simulink model "HANcoder_E407_TTA_Template_DS_V61"  (R2023a)
settings: Solver=FixedStepDiscrete  StartTime=0.0  StopTime=1  FixedStep=0.01  RelTol=1e-3
PreLoadFcn:
  | librarySetup
  | eval([bdroot,'_startup']) %Calling [modelName]_startup.m
values from neighbouring files (symbols this model uses):
  basic_cycle_duration_bc0 = TM_Reset_Board   + COMP_duration    (= 372)    [HANcoder_E407_TTA_Template_DS_V1_startup.m]    (also in HANcoder_E407_TTA_Template_DS_V2_startup.m; HANcoder_E407_TTA_Template_DS_V52_startup.m; HANcoder_E407_TTA_Template_DS_V5_startup.m; HANcoder_E407_TTA_Template_DS_V6_startup.m = 532)
  basic_cycle_duration_bc1 = basic_cycle_duration_bc0    (= 372)    [HANcoder_E407_TTA_Template_DS_V1_startup.m]    (also in HANcoder_E407_TTA_Template_DS_V2_startup.m; HANcoder_E407_TTA_Template_DS_V52_startup.m; HANcoder_E407_TTA_Template_DS_V5_startup.m; HANcoder_E407_TTA_Template_DS_V6_startup.m = 532)
  basic_cycle_duration_bc2 = basic_cycle_duration_bc0    (= 372)    [HANcoder_E407_TTA_Template_DS_V1_startup.m]    (also in HANcoder_E407_TTA_Template_DS_V2_startup.m; HANcoder_E407_TTA_Template_DS_V52_startup.m; HANcoder_E407_TTA_Template_DS_V5_startup.m; HANcoder_E407_TTA_Template_DS_V6_startup.m = 532)
  comm_delay_estimation1 = round(comm_delay_measured1*hardware_granularity/frequency_IRQ)    [HANcoder_E407_TTA_Template_DS_V1_startup.m]    (also in HANcoder_E407_TTA_Template_DS_V2_startup.m; HANcoder_E407_TTA_Template_DS_V52_startup.m; HANcoder_E407_TTA_Template_DS_V5_startup.m; HANcoder_E407_TTA_Template_DS_V6_startup.m)
  comm_delay_estimation2 = round(comm_delay_measured2*hardware_granularity/frequency_IRQ)    [HANcoder_E407_TTA_Template_DS_V1_startup.m]    (also in HANcoder_E407_TTA_Template_DS_V2_startup.m; HANcoder_E407_TTA_Template_DS_V52_startup.m; HANcoder_E407_TTA_Template_DS_V5_startup.m; HANcoder_E407_TTA_Template_DS_V6_startup.m)
  COMM_Period = 80    [HANcoder_E407_TTA_Template_DS_V1_startup.m]    (also in HANcoder_E407_TTA_Template_DS_V2_startup.m; HANcoder_E407_TTA_Template_DS_V52_startup.m; HANcoder_E407_TTA_Template_DS_V5_startup.m; HANcoder_E407_TTA_Template_DS_V6_startup.m = 120)
  COMM_Phase1 = Simulink.Parameter    [HANcoder_E407_TTA_Template_DS_V1_startup.m]    (also in HANcoder_E407_TTA_Template_DS_V2_startup.m; HANcoder_E407_TTA_Template_DS_V52_startup.m; HANcoder_E407_TTA_Template_DS_V5_startup.m; HANcoder_E407_TTA_Template_DS_V6_startup.m)
  COMM_Phase2 = Simulink.Parameter    [HANcoder_E407_TTA_Template_DS_V1_startup.m]    (also in HANcoder_E407_TTA_Template_DS_V2_startup.m; HANcoder_E407_TTA_Template_DS_V52_startup.m; HANcoder_E407_TTA_Template_DS_V5_startup.m; HANcoder_E407_TTA_Template_DS_V6_startup.m)
  COMM_Phase_init1 = Simulink.Parameter    [HANcoder_E407_TTA_Template_DS_V1_startup.m]    (also in HANcoder_E407_TTA_Template_DS_V2_startup.m; HANcoder_E407_TTA_Template_DS_V52_startup.m; HANcoder_E407_TTA_Template_DS_V5_startup.m; HANcoder_E407_TTA_Template_DS_V6_startup.m)
  COMM_Phase_init2 = Simulink.Parameter    [HANcoder_E407_TTA_Template_DS_V1_startup.m]    (also in HANcoder_E407_TTA_Template_DS_V2_startup.m; HANcoder_E407_TTA_Template_DS_V52_startup.m; HANcoder_E407_TTA_Template_DS_V5_startup.m; HANcoder_E407_TTA_Template_DS_V6_startup.m)
  COMP_duration = 4    [HANcoder_E407_TTA_Template_DS_V1_startup.m]    (also in HANcoder_E407_TTA_Template_DS_V2_startup.m; HANcoder_E407_TTA_Template_DS_V52_startup.m; HANcoder_E407_TTA_Template_DS_V5_startup.m; HANcoder_E407_TTA_Template_DS_V6_startup.m)
  frequency_IRQ = 100    [HANcoder_E407_TTA_Template_DS_V1_startup.m]    (also in HANcoder_E407_TTA_Template_DS_V2_startup.m; HANcoder_E407_TTA_Template_DS_V52_startup.m; HANcoder_E407_TTA_Template_DS_V5_startup.m; HANcoder_E407_TTA_Template_DS_V6_startup.m)
  idle_time_init = basic_cycle_duration_bc0 + basic_cycle_duration_bc1    (= 744)    [HANcoder_E407_TTA_Template_DS_V1_startup.m]    (also in HANcoder_E407_TTA_Template_DS_V2_startup.m; HANcoder_E407_TTA_Template_DS_V52_startup.m = 1116; HANcoder_E407_TTA_Template_DS_V5_startup.m = 1116; HANcoder_E407_TTA_Template_DS_V6_startup.m = 1596)
  L0b = 0.5    [HANcoder_E407_TTA_Template_DS_V52_startup.m]    (also in HANcoder_E407_TTA_Template_DS_V5_startup.m; HANcoder_E407_TTA_Template_DS_V6_startup.m)
  L0f = 5    [HANcoder_E407_TTA_Template_DS_V52_startup.m]    (also in HANcoder_E407_TTA_Template_DS_V5_startup.m; HANcoder_E407_TTA_Template_DS_V6_startup.m)
  L1f = 6    [HANcoder_E407_TTA_Template_DS_V52_startup.m]    (also in HANcoder_E407_TTA_Template_DS_V5_startup.m; HANcoder_E407_TTA_Template_DS_V6_startup.m)
  LA_Clock_Gr = 1    [HANcoder_E407_TTA_Template_DS_V1_startup.m]    (also in HANcoder_E407_TTA_Template_DS_V2_startup.m; HANcoder_E407_TTA_Template_DS_V52_startup.m; HANcoder_E407_TTA_Template_DS_V5_startup.m; HANcoder_E407_TTA_Template_DS_V6_startup.m)
  LA_COMM_dly = 1    [HANcoder_E407_TTA_Template_DS_V1_startup.m]    (also in HANcoder_E407_TTA_Template_DS_V2_startup.m; HANcoder_E407_TTA_Template_DS_V52_startup.m; HANcoder_E407_TTA_Template_DS_V5_startup.m; HANcoder_E407_TTA_Template_DS_V6_startup.m)
  LA_COMM_Err = 1    [HANcoder_E407_TTA_Template_DS_V1_startup.m]    (also in HANcoder_E407_TTA_Template_DS_V2_startup.m; HANcoder_E407_TTA_Template_DS_V52_startup.m; HANcoder_E407_TTA_Template_DS_V5_startup.m; HANcoder_E407_TTA_Template_DS_V6_startup.m)
  LA_E_Desync = 1    [HANcoder_E407_TTA_Template_DS_V1_startup.m]    (also in HANcoder_E407_TTA_Template_DS_V2_startup.m; HANcoder_E407_TTA_Template_DS_V52_startup.m; HANcoder_E407_TTA_Template_DS_V5_startup.m; HANcoder_E407_TTA_Template_DS_V6_startup.m)
  LA_MEX_Flag = 1    [HANcoder_E407_TTA_Template_DS_V1_startup.m]    (also in HANcoder_E407_TTA_Template_DS_V2_startup.m; HANcoder_E407_TTA_Template_DS_V52_startup.m; HANcoder_E407_TTA_Template_DS_V5_startup.m; HANcoder_E407_TTA_Template_DS_V6_startup.m)
  LA_Task_Act = 1    [HANcoder_E407_TTA_Template_DS_V1_startup.m]    (also in HANcoder_E407_TTA_Template_DS_V2_startup.m; HANcoder_E407_TTA_Template_DS_V52_startup.m; HANcoder_E407_TTA_Template_DS_V5_startup.m; HANcoder_E407_TTA_Template_DS_V6_startup.m)
  Master_Role = 1    [HANcoder_E407_TTA_Template_DS_V1_startup.m]    (also in HANcoder_E407_TTA_Template_DS_V2_startup.m; HANcoder_E407_TTA_Template_DS_V52_startup.m; HANcoder_E407_TTA_Template_DS_V5_startup.m; HANcoder_E407_TTA_Template_DS_V6_startup.m)
  matrix_rows = 3    [HANcoder_E407_TTA_Template_DS_V1_startup.m]    (also in HANcoder_E407_TTA_Template_DS_V2_startup.m; HANcoder_E407_TTA_Template_DS_V52_startup.m; HANcoder_E407_TTA_Template_DS_V5_startup.m; HANcoder_E407_TTA_Template_DS_V6_startup.m)
  max_desync = 15    [HANcoder_E407_TTA_Template_DS_V1_startup.m]    (also in HANcoder_E407_TTA_Template_DS_V2_startup.m; HANcoder_E407_TTA_Template_DS_V52_startup.m; HANcoder_E407_TTA_Template_DS_V5_startup.m; HANcoder_E407_TTA_Template_DS_V6_startup.m)
  max_num_msgs_CAN1 = 2^Tx_bit_number-1    (= 7)    [HANcoder_E407_TTA_Template_DS_V1_startup.m]    (also in HANcoder_E407_TTA_Template_DS_V2_startup.m; HANcoder_E407_TTA_Template_DS_V52_startup.m; HANcoder_E407_TTA_Template_DS_V5_startup.m; HANcoder_E407_TTA_Template_DS_V6_startup.m)
  max_num_msgs_CAN2 = max_num_msgs_CAN1    (= 7)    [HANcoder_E407_TTA_Template_DS_V1_startup.m]    (also in HANcoder_E407_TTA_Template_DS_V2_startup.m; HANcoder_E407_TTA_Template_DS_V52_startup.m; HANcoder_E407_TTA_Template_DS_V5_startup.m; HANcoder_E407_TTA_Template_DS_V6_startup.m)
  min_desync = (-1)*max_desync    (= -15)    [HANcoder_E407_TTA_Template_DS_V1_startup.m]    (also in HANcoder_E407_TTA_Template_DS_V2_startup.m; HANcoder_E407_TTA_Template_DS_V52_startup.m; HANcoder_E407_TTA_Template_DS_V5_startup.m; HANcoder_E407_TTA_Template_DS_V6_startup.m)
  PID_derivative = Simulink.Parameter    [HANcoder_E407_TTA_Template_DS_V52_startup.m]    (also in HANcoder_E407_TTA_Template_DS_V6_startup.m)
  PID_gain = Simulink.Parameter    [HANcoder_E407_TTA_Template_DS_V52_startup.m]    (also in HANcoder_E407_TTA_Template_DS_V6_startup.m)
  PID_integrator = Simulink.Parameter    [HANcoder_E407_TTA_Template_DS_V52_startup.m]    (also in HANcoder_E407_TTA_Template_DS_V6_startup.m)
  PotValue1_ID = 22    [HANcoder_E407_TTA_Template_DS_V1_startup.m]    (also in HANcoder_E407_TTA_Template_DS_V2_startup.m; HANcoder_E407_TTA_Template_DS_V52_startup.m; HANcoder_E407_TTA_Template_DS_V5_startup.m; HANcoder_E407_TTA_Template_DS_V6_startup.m)
  PotValue2_ID = 23    [HANcoder_E407_TTA_Template_DS_V1_startup.m]    (also in HANcoder_E407_TTA_Template_DS_V2_startup.m; HANcoder_E407_TTA_Template_DS_V52_startup.m; HANcoder_E407_TTA_Template_DS_V5_startup.m; HANcoder_E407_TTA_Template_DS_V6_startup.m)
  PotValue3_ID = 24    [HANcoder_E407_TTA_Template_DS_V1_startup.m]    (also in HANcoder_E407_TTA_Template_DS_V2_startup.m; HANcoder_E407_TTA_Template_DS_V52_startup.m; HANcoder_E407_TTA_Template_DS_V5_startup.m; HANcoder_E407_TTA_Template_DS_V6_startup.m)
  script_run = Simulink.Parameter    [HANcoder_E407_TTA_Template_DS_V1_startup.m]    (also in HANcoder_E407_TTA_Template_DS_V2_startup.m; HANcoder_E407_TTA_Template_DS_V52_startup.m; HANcoder_E407_TTA_Template_DS_V5_startup.m; HANcoder_E407_TTA_Template_DS_V6_startup.m)
  Slave_Role = 2    [HANcoder_E407_TTA_Template_DS_V1_startup.m]    (also in HANcoder_E407_TTA_Template_DS_V2_startup.m; HANcoder_E407_TTA_Template_DS_V52_startup.m; HANcoder_E407_TTA_Template_DS_V5_startup.m; HANcoder_E407_TTA_Template_DS_V6_startup.m)
  Sync_ID = 1    [HANcoder_E407_TTA_Template_DS_V1_startup.m]    (also in HANcoder_E407_TTA_Template_DS_V2_startup.m; HANcoder_E407_TTA_Template_DS_V52_startup.m; HANcoder_E407_TTA_Template_DS_V5_startup.m; HANcoder_E407_TTA_Template_DS_V6_startup.m)
  TM_Check_PotValue1 = TM_COMM_PotValue1 + COMM_duration    (= 174)    [HANcoder_E407_TTA_Template_DS_V1_startup.m]    (also in HANcoder_E407_TTA_Template_DS_V2_startup.m; HANcoder_E407_TTA_Template_DS_V52_startup.m; HANcoder_E407_TTA_Template_DS_V5_startup.m; HANcoder_E407_TTA_Template_DS_V6_startup.m = 254)
  TM_Check_PotValue2 = TM_COMM_PotValue2 + COMM_duration    (= 258)    [HANcoder_E407_TTA_Template_DS_V1_startup.m]    (also in HANcoder_E407_TTA_Template_DS_V2_startup.m; HANcoder_E407_TTA_Template_DS_V52_startup.m; HANcoder_E407_TTA_Template_DS_V5_startup.m; HANcoder_E407_TTA_Template_DS_V6_startup.m = 378)
  TM_Check_PotValue3 = TM_COMM_PotValue3 + COMM_duration    (= 342)    [HANcoder_E407_TTA_Template_DS_V1_startup.m]    (also in HANcoder_E407_TTA_Template_DS_V2_startup.m; HANcoder_E407_TTA_Template_DS_V52_startup.m; HANcoder_E407_TTA_Template_DS_V5_startup.m; HANcoder_E407_TTA_Template_DS_V6_startup.m = 502)
  TM_Check_Sync = TM_COMM_Sync   + COMM_duration    (= 80)    [HANcoder_E407_TTA_Template_DS_V1_startup.m]    (also in HANcoder_E407_TTA_Template_DS_V2_startup.m; HANcoder_E407_TTA_Template_DS_V52_startup.m; HANcoder_E407_TTA_Template_DS_V5_startup.m; HANcoder_E407_TTA_Template_DS_V6_startup.m = 120)
  TM_Check_TOuts = TM_Count_Vote3 + COMP_duration    (= 356)    [HANcoder_E407_TTA_Template_DS_V1_startup.m]    (also in HANcoder_E407_TTA_Template_DS_V2_startup.m; HANcoder_E407_TTA_Template_DS_V52_startup.m; HANcoder_E407_TTA_Template_DS_V5_startup.m; HANcoder_E407_TTA_Template_DS_V6_startup.m = 516)
  TM_Check_Trailer1Articulation = TM_COMM_Trailer1Articulation + COMM_duration    (= 170)    [HANcoder_E407_TTA_Template_DS_V1_startup.m]    (also in HANcoder_E407_TTA_Template_DS_V2_startup.m; HANcoder_E407_TTA_Template_DS_V52_startup.m; HANcoder_E407_TTA_Template_DS_V5_startup.m; HANcoder_E407_TTA_Template_DS_V6_startup.m = 250)
  TM_Check_Trailer2Articulation = TM_COMM_Trailer2Articulation + COMM_duration    (= 254)    [HANcoder_E407_TTA_Template_DS_V1_startup.m]    (also in HANcoder_E407_TTA_Template_DS_V2_startup.m; HANcoder_E407_TTA_Template_DS_V52_startup.m; HANcoder_E407_TTA_Template_DS_V5_startup.m; HANcoder_E407_TTA_Template_DS_V6_startup.m = 374)
  TM_Check_Vote1 = TM_COMM_Vote1  + COMM_duration    (= 172)    [HANcoder_E407_TTA_Template_DS_V1_startup.m]    (also in HANcoder_E407_TTA_Template_DS_V2_startup.m; HANcoder_E407_TTA_Template_DS_V52_startup.m; HANcoder_E407_TTA_Template_DS_V5_startup.m; HANcoder_E407_TTA_Template_DS_V6_startup.m = 252)
  TM_Check_Vote2 = TM_COMM_Vote2  + COMM_duration    (= 260)    [HANcoder_E407_TTA_Template_DS_V1_startup.m]    (also in HANcoder_E407_TTA_Template_DS_V2_startup.m; HANcoder_E407_TTA_Template_DS_V52_startup.m; HANcoder_E407_TTA_Template_DS_V5_startup.m; HANcoder_E407_TTA_Template_DS_V6_startup.m = 380)
  TM_Check_Vote3 = TM_COMM_Vote3  + COMM_duration    (= 348)    [HANcoder_E407_TTA_Template_DS_V1_startup.m]    (also in HANcoder_E407_TTA_Template_DS_V2_startup.m; HANcoder_E407_TTA_Template_DS_V52_startup.m; HANcoder_E407_TTA_Template_DS_V5_startup.m; HANcoder_E407_TTA_Template_DS_V6_startup.m = 508)
  TM_COMM_PotValue1 = TM_ReadPot + COMP_duration    (= 94)    [HANcoder_E407_TTA_Template_DS_V1_startup.m]    (also in HANcoder_E407_TTA_Template_DS_V2_startup.m; HANcoder_E407_TTA_Template_DS_V52_startup.m; HANcoder_E407_TTA_Template_DS_V5_startup.m; HANcoder_E407_TTA_Template_DS_V6_startup.m = 134)
  TM_COMM_PotValue2 = TM_Check_PotValue1 + COMP_duration    (= 178)    [HANcoder_E407_TTA_Template_DS_V1_startup.m]    (also in HANcoder_E407_TTA_Template_DS_V2_startup.m; HANcoder_E407_TTA_Template_DS_V52_startup.m; HANcoder_E407_TTA_Template_DS_V5_startup.m; HANcoder_E407_TTA_Template_DS_V6_startup.m = 258)
  TM_COMM_PotValue3 = TM_Check_PotValue2 + COMP_duration    (= 262)    [HANcoder_E407_TTA_Template_DS_V1_startup.m]    (also in HANcoder_E407_TTA_Template_DS_V2_startup.m; HANcoder_E407_TTA_Template_DS_V52_startup.m; HANcoder_E407_TTA_Template_DS_V5_startup.m; HANcoder_E407_TTA_Template_DS_V6_startup.m = 382)
  TM_COMM_Sync = basic_cycle_start    (= 0)    [HANcoder_E407_TTA_Template_DS_V1_startup.m]    (also in HANcoder_E407_TTA_Template_DS_V2_startup.m; HANcoder_E407_TTA_Template_DS_V52_startup.m; HANcoder_E407_TTA_Template_DS_V5_startup.m; HANcoder_E407_TTA_Template_DS_V6_startup.m)
  TM_COMM_Trailer1Articulation = TM_Update_LT_2 + COMP_duration    (= 90)    [HANcoder_E407_TTA_Template_DS_V1_startup.m]    (also in HANcoder_E407_TTA_Template_DS_V2_startup.m; HANcoder_E407_TTA_Template_DS_V52_startup.m; HANcoder_E407_TTA_Template_DS_V5_startup.m; HANcoder_E407_TTA_Template_DS_V6_startup.m = 130)
  TM_COMM_Trailer2Articulation = TM_Check_Trailer1Articulation + COMP_duration    (= 174)    [HANcoder_E407_TTA_Template_DS_V1_startup.m]    (also in HANcoder_E407_TTA_Template_DS_V2_startup.m; HANcoder_E407_TTA_Template_DS_V52_startup.m; HANcoder_E407_TTA_Template_DS_V5_startup.m; HANcoder_E407_TTA_Template_DS_V6_startup.m = 254)
  TM_COMM_Vote1 = TM_Vote_Dec    + COMP_duration    (= 92)    [HANcoder_E407_TTA_Template_DS_V1_startup.m]    (also in HANcoder_E407_TTA_Template_DS_V2_startup.m; HANcoder_E407_TTA_Template_DS_V52_startup.m; HANcoder_E407_TTA_Template_DS_V5_startup.m; HANcoder_E407_TTA_Template_DS_V6_startup.m = 132)
  TM_COMM_Vote2 = TM_Count_Vote1 + COMP_duration    (= 180)    [HANcoder_E407_TTA_Template_DS_V1_startup.m]    (also in HANcoder_E407_TTA_Template_DS_V2_startup.m; HANcoder_E407_TTA_Template_DS_V52_startup.m; HANcoder_E407_TTA_Template_DS_V5_startup.m; HANcoder_E407_TTA_Template_DS_V6_startup.m = 260)
  TM_COMM_Vote3 = TM_Count_Vote2 + COMP_duration    (= 268)    [HANcoder_E407_TTA_Template_DS_V1_startup.m]    (also in HANcoder_E407_TTA_Template_DS_V2_startup.m; HANcoder_E407_TTA_Template_DS_V52_startup.m; HANcoder_E407_TTA_Template_DS_V5_startup.m; HANcoder_E407_TTA_Template_DS_V6_startup.m = 388)
  TM_Count_Vote1 = TM_Check_Vote1 + COMP_duration    (= 176)    [HANcoder_E407_TTA_Template_DS_V1_startup.m]    (also in HANcoder_E407_TTA_Template_DS_V2_startup.m; HANcoder_E407_TTA_Template_DS_V52_startup.m; HANcoder_E407_TTA_Template_DS_V5_startup.m; HANcoder_E407_TTA_Template_DS_V6_startup.m = 256)
  TM_Count_Vote2 = TM_Check_Vote2 + COMP_duration    (= 264)    [HANcoder_E407_TTA_Template_DS_V1_startup.m]    (also in HANcoder_E407_TTA_Template_DS_V2_startup.m; HANcoder_E407_TTA_Template_DS_V52_startup.m; HANcoder_E407_TTA_Template_DS_V5_startup.m; HANcoder_E407_TTA_Template_DS_V6_startup.m = 384)
  TM_Count_Vote3 = TM_Check_Vote3 + COMP_duration    (= 352)    [HANcoder_E407_TTA_Template_DS_V1_startup.m]    (also in HANcoder_E407_TTA_Template_DS_V2_startup.m; HANcoder_E407_TTA_Template_DS_V52_startup.m; HANcoder_E407_TTA_Template_DS_V5_startup.m; HANcoder_E407_TTA_Template_DS_V6_startup.m = 512)
  TM_Data_bc0 = TM_COMM_Sync    (= 0)    [HANcoder_E407_TTA_Template_DS_V1_startup.m]    (also in HANcoder_E407_TTA_Template_DS_V2_startup.m; HANcoder_E407_TTA_Template_DS_V52_startup.m; HANcoder_E407_TTA_Template_DS_V5_startup.m; HANcoder_E407_TTA_Template_DS_V6_startup.m)
  TM_Data_bc1 = TM_Data_bc0(1:4)    [HANcoder_E407_TTA_Template_DS_V1_startup.m]    (also in HANcoder_E407_TTA_Template_DS_V2_startup.m; HANcoder_E407_TTA_Template_DS_V52_startup.m; HANcoder_E407_TTA_Template_DS_V5_startup.m; HANcoder_E407_TTA_Template_DS_V6_startup.m)
  TM_Data_bc2 = TM_Data_bc0(1:4)    [HANcoder_E407_TTA_Template_DS_V1_startup.m]    (also in HANcoder_E407_TTA_Template_DS_V2_startup.m; HANcoder_E407_TTA_Template_DS_V52_startup.m; HANcoder_E407_TTA_Template_DS_V5_startup.m; HANcoder_E407_TTA_Template_DS_V6_startup.m)
  TM_InverseKinematics = TM_Check_Trailer2Articulation + COMP_duration    (= 258)    [HANcoder_E407_TTA_Template_DS_V1_startup.m]    (also in HANcoder_E407_TTA_Template_DS_V2_startup.m; HANcoder_E407_TTA_Template_DS_V52_startup.m; HANcoder_E407_TTA_Template_DS_V5_startup.m; HANcoder_E407_TTA_Template_DS_V6_startup.m = 378)
  TM_New_Master = TM_Check_TOuts + COMP_duration    (= 360)    [HANcoder_E407_TTA_Template_DS_V1_startup.m]    (also in HANcoder_E407_TTA_Template_DS_V2_startup.m; HANcoder_E407_TTA_Template_DS_V52_startup.m; HANcoder_E407_TTA_Template_DS_V5_startup.m; HANcoder_E407_TTA_Template_DS_V6_startup.m = 520)
  TM_PotVote = TM_COMM_PotValue3 + COMP_duration    (= 266)    [HANcoder_E407_TTA_Template_DS_V1_startup.m]    (also in HANcoder_E407_TTA_Template_DS_V2_startup.m; HANcoder_E407_TTA_Template_DS_V52_startup.m; HANcoder_E407_TTA_Template_DS_V5_startup.m; HANcoder_E407_TTA_Template_DS_V6_startup.m = 386)
  TM_ReadPot = TM_Update_LT_2 + COMP_duration    (= 90)    [HANcoder_E407_TTA_Template_DS_V1_startup.m]    (also in HANcoder_E407_TTA_Template_DS_V2_startup.m; HANcoder_E407_TTA_Template_DS_V52_startup.m; HANcoder_E407_TTA_Template_DS_V5_startup.m; HANcoder_E407_TTA_Template_DS_V6_startup.m = 130)
  TM_Reset_Board = TM_Reset_Var   + COMP_duration    (= 368)    [HANcoder_E407_TTA_Template_DS_V1_startup.m]    (also in HANcoder_E407_TTA_Template_DS_V2_startup.m; HANcoder_E407_TTA_Template_DS_V52_startup.m; HANcoder_E407_TTA_Template_DS_V5_startup.m; HANcoder_E407_TTA_Template_DS_V6_startup.m = 528)
  TM_Reset_Var = TM_New_Master  + COMP_duration    (= 364)    [HANcoder_E407_TTA_Template_DS_V1_startup.m]    (also in HANcoder_E407_TTA_Template_DS_V2_startup.m; HANcoder_E407_TTA_Template_DS_V52_startup.m; HANcoder_E407_TTA_Template_DS_V5_startup.m; HANcoder_E407_TTA_Template_DS_V6_startup.m = 524)
  TM_Reset_Var_bc1 = TM_Data_bc1(end) + COMP_duration    [HANcoder_E407_TTA_Template_DS_V1_startup.m]    (also in HANcoder_E407_TTA_Template_DS_V2_startup.m; HANcoder_E407_TTA_Template_DS_V52_startup.m; HANcoder_E407_TTA_Template_DS_V5_startup.m; HANcoder_E407_TTA_Template_DS_V6_startup.m)
  TM_Reset_Var_bc1_2 = TM_Reset_Var_bc1 +2    [HANcoder_E407_TTA_Template_DS_V1_startup.m]    (also in HANcoder_E407_TTA_Template_DS_V2_startup.m; HANcoder_E407_TTA_Template_DS_V52_startup.m; HANcoder_E407_TTA_Template_DS_V5_startup.m; HANcoder_E407_TTA_Template_DS_V6_startup.m)
  TM_Reset_Var_bc2 = TM_Data_bc2(end) + COMP_duration    [HANcoder_E407_TTA_Template_DS_V1_startup.m]    (also in HANcoder_E407_TTA_Template_DS_V2_startup.m; HANcoder_E407_TTA_Template_DS_V52_startup.m; HANcoder_E407_TTA_Template_DS_V5_startup.m; HANcoder_E407_TTA_Template_DS_V6_startup.m)
  TM_Reset_Var_bc2_2 = TM_Reset_Var_bc2 +2    [HANcoder_E407_TTA_Template_DS_V1_startup.m]    (also in HANcoder_E407_TTA_Template_DS_V2_startup.m; HANcoder_E407_TTA_Template_DS_V52_startup.m; HANcoder_E407_TTA_Template_DS_V5_startup.m; HANcoder_E407_TTA_Template_DS_V6_startup.m)
  TM_Type_bc0 = COMM    (= 0)    [HANcoder_E407_TTA_Template_DS_V1_startup.m]    (also in HANcoder_E407_TTA_Template_DS_V2_startup.m; HANcoder_E407_TTA_Template_DS_V52_startup.m; HANcoder_E407_TTA_Template_DS_V5_startup.m; HANcoder_E407_TTA_Template_DS_V6_startup.m)
  TM_Type_bc1 = TM_Type_bc0(1:4)    [HANcoder_E407_TTA_Template_DS_V1_startup.m]    (also in HANcoder_E407_TTA_Template_DS_V2_startup.m; HANcoder_E407_TTA_Template_DS_V52_startup.m; HANcoder_E407_TTA_Template_DS_V5_startup.m; HANcoder_E407_TTA_Template_DS_V6_startup.m)
  TM_Type_bc2 = TM_Type_bc0(1:4)    [HANcoder_E407_TTA_Template_DS_V1_startup.m]    (also in HANcoder_E407_TTA_Template_DS_V2_startup.m; HANcoder_E407_TTA_Template_DS_V52_startup.m; HANcoder_E407_TTA_Template_DS_V5_startup.m; HANcoder_E407_TTA_Template_DS_V6_startup.m)
  TM_Update_LT = TM_Check_Sync  + COMP_duration    (= 84)    [HANcoder_E407_TTA_Template_DS_V1_startup.m]    (also in HANcoder_E407_TTA_Template_DS_V2_startup.m; HANcoder_E407_TTA_Template_DS_V52_startup.m; HANcoder_E407_TTA_Template_DS_V5_startup.m; HANcoder_E407_TTA_Template_DS_V6_startup.m = 124)
  TM_Update_LT_2 = TM_Update_LT   + 2    (= 86)    [HANcoder_E407_TTA_Template_DS_V1_startup.m]    (also in HANcoder_E407_TTA_Template_DS_V2_startup.m; HANcoder_E407_TTA_Template_DS_V52_startup.m; HANcoder_E407_TTA_Template_DS_V5_startup.m; HANcoder_E407_TTA_Template_DS_V6_startup.m = 126)
  TM_Vote_Dec = TM_Update_LT   + COMP_duration    (= 88)    [HANcoder_E407_TTA_Template_DS_V1_startup.m]    (also in HANcoder_E407_TTA_Template_DS_V2_startup.m; HANcoder_E407_TTA_Template_DS_V52_startup.m; HANcoder_E407_TTA_Template_DS_V5_startup.m; HANcoder_E407_TTA_Template_DS_V6_startup.m = 128)
  Tractor_Board1 = 11    [HANcoder_E407_TTA_Template_DS_V1_startup.m]    (also in HANcoder_E407_TTA_Template_DS_V2_startup.m = 1; HANcoder_E407_TTA_Template_DS_V52_startup.m = 1; HANcoder_E407_TTA_Template_DS_V5_startup.m = 1; HANcoder_E407_TTA_Template_DS_V6_startup.m = 1)
  Tractor_Board2 = 12    [HANcoder_E407_TTA_Template_DS_V1_startup.m]    (also in HANcoder_E407_TTA_Template_DS_V2_startup.m = 2; HANcoder_E407_TTA_Template_DS_V52_startup.m = 2; HANcoder_E407_TTA_Template_DS_V5_startup.m = 2; HANcoder_E407_TTA_Template_DS_V6_startup.m = 2)
  Tractor_Board3 = 13    [HANcoder_E407_TTA_Template_DS_V1_startup.m]    (also in HANcoder_E407_TTA_Template_DS_V2_startup.m = 3; HANcoder_E407_TTA_Template_DS_V52_startup.m = 3; HANcoder_E407_TTA_Template_DS_V5_startup.m = 3; HANcoder_E407_TTA_Template_DS_V6_startup.m = 3)
  Trailer1_Articulation_ID = 31    [HANcoder_E407_TTA_Template_DS_V1_startup.m]    (also in HANcoder_E407_TTA_Template_DS_V2_startup.m; HANcoder_E407_TTA_Template_DS_V52_startup.m; HANcoder_E407_TTA_Template_DS_V5_startup.m; HANcoder_E407_TTA_Template_DS_V6_startup.m)
  Trailer1_Board1 = 2    [HANcoder_E407_TTA_Template_DS_V1_startup.m]    (also in HANcoder_E407_TTA_Template_DS_V2_startup.m = 4; HANcoder_E407_TTA_Template_DS_V52_startup.m = 4; HANcoder_E407_TTA_Template_DS_V5_startup.m = 4; HANcoder_E407_TTA_Template_DS_V6_startup.m = 4)
  Trailer1_Board2 = 3    [HANcoder_E407_TTA_Template_DS_V1_startup.m]    (also in HANcoder_E407_TTA_Template_DS_V2_startup.m = 5; HANcoder_E407_TTA_Template_DS_V52_startup.m = 5; HANcoder_E407_TTA_Template_DS_V5_startup.m = 5; HANcoder_E407_TTA_Template_DS_V6_startup.m = 5)
  Trailer1_Board3 = 4    [HANcoder_E407_TTA_Template_DS_V1_startup.m]    (also in HANcoder_E407_TTA_Template_DS_V2_startup.m = 6; HANcoder_E407_TTA_Template_DS_V52_startup.m = 6; HANcoder_E407_TTA_Template_DS_V5_startup.m = 6; HANcoder_E407_TTA_Template_DS_V6_startup.m = 6)
  Trailer2_Articulation_ID = 32    [HANcoder_E407_TTA_Template_DS_V1_startup.m]    (also in HANcoder_E407_TTA_Template_DS_V2_startup.m; HANcoder_E407_TTA_Template_DS_V52_startup.m; HANcoder_E407_TTA_Template_DS_V5_startup.m; HANcoder_E407_TTA_Template_DS_V6_startup.m)
  Trailer2_Board1 = 5    [HANcoder_E407_TTA_Template_DS_V1_startup.m]    (also in HANcoder_E407_TTA_Template_DS_V2_startup.m = 7; HANcoder_E407_TTA_Template_DS_V52_startup.m = 7; HANcoder_E407_TTA_Template_DS_V5_startup.m = 7; HANcoder_E407_TTA_Template_DS_V6_startup.m = 7)
  Trailer2_Board2 = 6    [HANcoder_E407_TTA_Template_DS_V1_startup.m]    (also in HANcoder_E407_TTA_Template_DS_V2_startup.m = 8; HANcoder_E407_TTA_Template_DS_V52_startup.m = 8; HANcoder_E407_TTA_Template_DS_V5_startup.m = 8; HANcoder_E407_TTA_Template_DS_V6_startup.m = 8)
  Trailer2_Board3 = 7    [HANcoder_E407_TTA_Template_DS_V1_startup.m]    (also in HANcoder_E407_TTA_Template_DS_V2_startup.m = 9; HANcoder_E407_TTA_Template_DS_V52_startup.m = 9; HANcoder_E407_TTA_Template_DS_V5_startup.m = 9; HANcoder_E407_TTA_Template_DS_V6_startup.m = 9)
  V1 = -0.000000001    (= -1e-09)    [HANcoder_E407_TTA_Template_DS_V52_startup.m]    (also in HANcoder_E407_TTA_Template_DS_V5_startup.m; HANcoder_E407_TTA_Template_DS_V6_startup.m)
  V2 = -0.000000001    (= -1e-09)    [HANcoder_E407_TTA_Template_DS_V52_startup.m]    (also in HANcoder_E407_TTA_Template_DS_V5_startup.m; HANcoder_E407_TTA_Template_DS_V6_startup.m)
  Vote1_ID = 11    [HANcoder_E407_TTA_Template_DS_V1_startup.m]    (also in HANcoder_E407_TTA_Template_DS_V2_startup.m; HANcoder_E407_TTA_Template_DS_V52_startup.m; HANcoder_E407_TTA_Template_DS_V5_startup.m; HANcoder_E407_TTA_Template_DS_V6_startup.m)
  Vote2_ID = 12    [HANcoder_E407_TTA_Template_DS_V1_startup.m]    (also in HANcoder_E407_TTA_Template_DS_V2_startup.m; HANcoder_E407_TTA_Template_DS_V52_startup.m; HANcoder_E407_TTA_Template_DS_V5_startup.m; HANcoder_E407_TTA_Template_DS_V6_startup.m)
  Vote3_ID = 13    [HANcoder_E407_TTA_Template_DS_V1_startup.m]    (also in HANcoder_E407_TTA_Template_DS_V2_startup.m; HANcoder_E407_TTA_Template_DS_V52_startup.m; HANcoder_E407_TTA_Template_DS_V5_startup.m; HANcoder_E407_TTA_Template_DS_V6_startup.m)
undefined symbols (not defined in the file or in its folder): A0, A1, A2, A3, A4, A5, CON2, CON3, CON4, D10, D12, D13, D6, D7, D8, D9
libraries: hdlsllib x136, simulink x39, HANcoder_STM32_Target x31, simulink_extras x8, dspstat3 x2, slpidlib x1
(part 15 of 42)

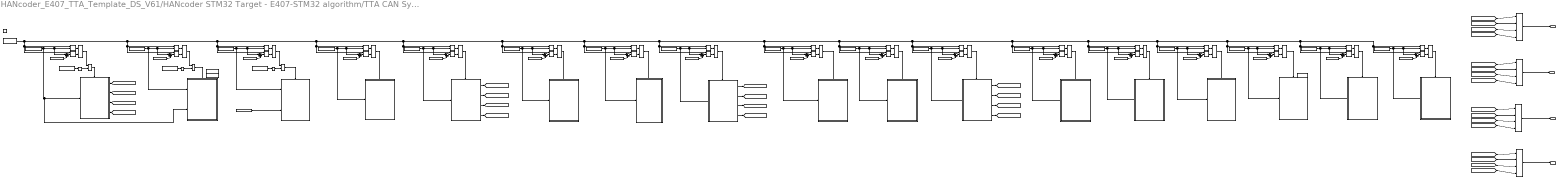
== system HANcoder_E407_TTA_Template_DS_V61/HANcoder STM32 Target - E407-STM32 algorithm/TTA CAN System/TTA System/Matrix Cycle Manager/Controller Matrix Cycle/controller basic cycle 0 ==
  note: Output Send_Message
      | Send: 1
      | Do not send: 0
  note: Send message condition
      | Sync Msg: Master and TM0
      | Vote Msg: Node# and TM#
  note: Receive message condition
      | Sync Msg: Not Master and TM0
      | Vote Msg: Not # Node at TM#
  note: Receive message condition
      | Sync Msg: Not Master and TM0
      | Vote Msg: Not # Node at TM#
  note: Output Receive_Message
      | Receive: 1
      | Do not receive: 0
  note: Output Send_Message
      | Send: 1
      | Do not send: 0
  note: Output Receive_Message
      | Receive: 1
      | Do not receive: 0
  note: Send message condition
      | Sync Msg: Master and TM0
      | Vote Msg: Node# and TM#
  note: COMM - TW check
  note: COMP - TW check
  note: COMP - TW check
  note: COMP - TW check
  note: COMM - TW check
  note: COMP - TW check
  note: COMP - TW check
  note: COMM - TW check
  note: COMP - TW check
  note: COMP - TW check
  note: COMM - TW check
  note: COMP - TW check
  note: COMP - TW check
  note: COMP - TW check
  note: COMP - TW check
  note: COMP - TW check
  note: COMP - TW check
  note: Local Time still not updated
  note: Local Time still not updated
  note: Local Time still not updated
  Enable : EnablePort  PropagateVarSize=During execution
  AND{,1..19} (20 alike) : Logic  IconShape=distinctive  AllPortsSameDT=off  OutDataTypeStr=boolean
  COMM Task - Sync bc 0 : Subsystem
  COMM Task - Vote1 : Subsystem
  COMM Task - Vote2 : Subsystem
  COMM Task - Vote3 : Subsystem
  COMP Task - Check Timeouts : Subsystem
  COMP Task - New Master : Subsystem
  COMP Task - Reset Board : Subsystem
  COMP Task - Reset Variables BC0 : Subsystem
  COMP Task - Sync bc0 check : Subsystem
  COMP Task - Update LT : Subsystem
  COMP Task - Vote Decision : Subsystem
  COMP Task - Vote1 Count : Subsystem
  COMP Task - Vote1 check : Subsystem
  COMP Task - Vote2 Count : Subsystem
  COMP Task - Vote2 check : Subsystem
  COMP Task - Vote3 Count : Subsystem
  COMP Task - Vote3 check : Subsystem
  Constant : Constant  Value=TM_COMM_Sync
  Constant{1,4,10,29} (4 alike) : Constant  Value=COMM_Period
  Constant{5,7,11,13,15..16,18,20,22,24,26,30,32} (13 alike) : Constant  Value=COMP_duration
  Constant12 : Constant  Value=TM_Check_TOuts
  Constant14 : Constant  Value=TM_New_Master
  Constant17 : Constant  Value=TM_Update_LT
  Constant19 : Constant  Value=TM_Vote_Dec
  Constant2 : Constant  Value=TM_Check_Sync
  Constant21 : Constant  Value=TM_Count_Vote1
  Constant23 : Constant  Value=TM_Check_Vote3
  Constant25 : Constant  Value=TM_Reset_Var
  Constant27 : Constant  Value=TM_Count_Vote2
  Constant28 : Constant  Value=TM_COMM_Vote2
  Constant3 : Constant  Value=TM_COMM_Vote1
  Constant31 : Constant  Value=TM_Reset_Board
  Constant33 : Constant  Value=TM_Check_Vote2
  Constant34 : Constant  Value=TM_Update_LT_2
  Constant6 : Constant  Value=TM_Check_Vote1
  Constant8 : Constant  Value=TM_Count_Vote3
  Constant9 : Constant  Value=TM_COMM_Vote3
  Data Store Memory11 : DataStoreMemory  DataStoreName=Msg_Rx  ReadBeforeWriteMsg=warning  WriteAfterWriteMsg=warning  WriteAfterReadMsg=warning  ShowAdditionalParam=off  OutDataTypeStr=Bus: msg_buffer_type
  Data Store Memory7 : DataStoreMemory  DataStoreName=Reset_Board  ReadBeforeWriteMsg=warning  WriteAfterWriteMsg=warning  WriteAfterReadMsg=warning  ShowAdditionalParam=off  OutDataTypeStr=boolean
  Data Store Memory8 : DataStoreMemory  DataStoreName=new_msg_Rx  ReadBeforeWriteMsg=warning  WriteAfterWriteMsg=warning  WriteAfterReadMsg=warning  ShowAdditionalParam=off
  Data Store Read11 : DataStoreRead  DataStoreName=BC0_Sync_processed  IndexOptions=Index vector (dialog)  Indices=1  OutputSizes=1
  Data Store Read6 : DataStoreRead  DataStoreName=BC0_Sync_processed  IndexOptions=Index vector (dialog)  Indices=1  OutputSizes=1
  Data Store Read7 : DataStoreRead  DataStoreName=BC0_Sync_processed  IndexOptions=Index vector (dialog)  Indices=1  OutputSizes=1
  Data Store Read8 : DataStoreRead  DataStoreName=Local_Ticks  IndexOptions=Index vector (dialog)  Indices=1  OutputSizes=1
  GreaterThan{,2,4,6,8,10,12,14,16,18,20,22,24,26,28,30,32} (17 alike) : RelationalOperator  OutDataTypeStr=boolean  RndMeth=Simplest  InputSameDT=off
  GreaterThan{1,3,5,7,9,11,13,15,17,19,21,23,25,27,29,31,33} (17 alike) : RelationalOperator  Operator=<  OutDataTypeStr=boolean  RndMeth=Simplest  InputSameDT=off
  NOT1 : Logic  Operator=NOT  IconShape=distinctive  AllPortsSameDT=off  OutDataTypeStr=boolean
  NOT2 : Logic  Operator=NOT  IconShape=distinctive  AllPortsSameDT=off  OutDataTypeStr=boolean
  NOT3 : Logic  Operator=NOT  IconShape=distinctive  AllPortsSameDT=off  OutDataTypeStr=boolean
  OR{1..4} (4 alike) : Logic  Operator=OR  Inputs=4  IconShape=distinctive  AllPortsSameDT=off  OutDataTypeStr=boolean
  Sum{1..17} (17 alike) : Sum  Inputs=|++
  Send_Message_CAN1 : Outport  OutputWhenDisabled=reset  InitialOutput=0  VectorParamsAs1DForOutWhenUnconnected=off
  Send_Message_CAN2 : Outport  Port=2  OutputWhenDisabled=reset  InitialOutput=0  VectorParamsAs1DForOutWhenUnconnected=off
  Receive_Message_CAN1 : Outport  Port=3  OutputWhenDisabled=reset  InitialOutput=0  VectorParamsAs1DForOutWhenUnconnected=off
  Receive_Message_CAN2 : Outport  Port=4  OutputWhenDisabled=reset  InitialOutput=0  VectorParamsAs1DForOutWhenUnconnected=off
  wires:
  OR1/1 -> Send_Message_CAN1/1
  [receive_CAN2_Sync_bc0_TAG] -> OR3/1
  [receive_CAN2_Vote3_bc0_TAG] -> OR3/4
  [receive_CAN2_Vote1_bc0_TAG] -> OR3/2
  [receive_CAN2_Vote2_bc0_TAG] -> OR3/3
  OR3/1 -> Receive_Message_CAN2/1
  [receive_CAN1_Sync_bc0_TAG] -> OR2/1
  [receive_CAN1_Vote1_bc0_TAG] -> OR2/2
  [receive_CAN1_Vote2_bc0_TAG] -> OR2/3
  [receive_CAN1_Vote3_bc0_TAG] -> OR2/4
  OR2/1 -> Receive_Message_CAN1/1
  [send_CAN2_Sync_bc0_TAG] -> OR4/1
  [send_CAN2_Vote1_bc0_TAG] -> OR4/2
  [send_CAN2_Vote2_bc0_TAG] -> OR4/3
  [send_CAN2_Vote3_bc0_TAG] -> OR4/4
  [send_CAN1_Sync_bc0_TAG] -> OR1/1
  [send_CAN1_Vote1_bc0_TAG] -> OR1/2
  [send_CAN1_Vote2_bc0_TAG] -> OR1/3
  [send_CAN1_Vote3_bc0_TAG] -> OR1/4
  OR4/1 -> Send_Message_CAN2/1
  COMM Task - Sync bc 0/1(Send CAN1) -> [send_CAN1_Sync_bc0_TAG]
  COMM Task - Sync bc 0/2(Receive CAN1) -> [receive_CAN1_Sync_bc0_TAG]
  COMM Task - Sync bc 0/3(Send CAN2) -> [send_CAN2_Sync_bc0_TAG]
  COMM Task - Sync bc 0/4(Receive CAN2) -> [receive_CAN2_Sync_bc0_TAG]
  Constant1/1 -> Sum4/2
  Constant/1 -> COMP Task - Sync bc0 check/2(TM_COMM), COMM Task - Sync bc 0/1(Time Mark), Sum4/1, GreaterThan/2
  Sum4/1 -> GreaterThan1/2
  GreaterThan/1 -> AND/1
  GreaterThan1/1 -> AND/2
  AND/1 -> AND17/1
  GreaterThan3/1 -> AND1/2
  GreaterThan2/1 -> AND1/1
  Sum1/1 -> GreaterThan3/2
  Constant2/1 -> COMP Task - Sync bc0 check/1(Time_Mark), GreaterThan2/2, Sum1/1
  Constant15/1 -> Sum1/2
  Constant16/1 -> Sum2/2
  Constant17/1 -> COMP Task - Update LT/1(Time_Mark), Sum2/1, GreaterThan4/2
  Sum2/1 -> GreaterThan5/2
  GreaterThan4/1 -> AND2/1
  GreaterThan5/1 -> AND2/2
  AND3/1 -> COMP Task - Vote Decision/Enable
  GreaterThan7/1 -> AND3/2
  GreaterThan6/1 -> AND3/1
  Sum3/1 -> GreaterThan7/2
  Constant19/1 -> COMP Task - Vote Decision/1(Time Mark), GreaterThan6/2, Sum3/1
  Constant18/1 -> Sum3/2
  COMM Task - Vote1/1(Send CAN1) -> [send_CAN1_Vote1_bc0_TAG]
  COMM Task - Vote1/2(Receive CAN1) -> [receive_CAN1_Vote1_bc0_TAG]
  COMM Task - Vote1/3(Send CAN2) -> [send_CAN2_Vote1_bc0_TAG]
  COMM Task - Vote1/4(Receive CAN2) -> [receive_CAN2_Vote1_bc0_TAG]
  GreaterThan9/1 -> AND4/2
  GreaterThan8/1 -> AND4/1
  Sum5/1 -> GreaterThan9/2
  Constant4/1 -> Sum5/2
  AND4/1 -> COMM Task - Vote1/Enable
  Constant3/1 -> COMM Task - Vote1/1(Time Mark), Sum5/1, GreaterThan8/2
  GreaterThan11/1 -> AND5/2
  Sum6/1 -> GreaterThan11/2
  GreaterThan10/1 -> AND5/1
  Constant5/1 -> Sum6/2
  Constant6/1 -> COMP Task - Vote1 check/1(Time_Mark), GreaterThan10/2, Sum6/1
  AND5/1 -> COMP Task - Vote1 check/Enable
  AND6/1 -> COMP Task - Vote1 Count/Enable
  Constant21/1 -> COMP Task - Vote1 Count/1(Time Mark), Sum7/1, GreaterThan12/2
  Constant20/1 -> Sum7/2
  GreaterThan12/1 -> AND6/1
  Sum7/1 -> GreaterThan13/2
  GreaterThan13/1 -> AND6/2
  GreaterThan17/1 -> AND9/2
  Sum10/1 -> GreaterThan17/2
  GreaterThan16/1 -> AND9/1
  Constant26/1 -> Sum10/2
  Constant27/1 -> COMP Task - Vote2 Count/1(Time Mark), GreaterThan16/2, Sum10/1
  AND9/1 -> COMP Task - Vote2 Count/Enable
  Constant33/1 -> COMP Task - Vote2 check/1(Time_Mark), Sum9/1, GreaterThan14/2
  Constant32/1 -> Sum9/2
  GreaterThan14/1 -> AND8/1
  Sum9/1 -> GreaterThan15/2
  GreaterThan15/1 -> AND8/2
  Constant28/1 -> COMM Task - Vote2/1(Time Mark), GreaterThan18/2, Sum8/1
  AND7/1 -> COMM Task - Vote2/Enable
  Constant29/1 -> Sum8/2
  Sum8/1 -> GreaterThan19/2
  GreaterThan18/1 -> AND7/1
  GreaterThan19/1 -> AND7/2
  COMM Task - Vote2/1(Send CAN1) -> [send_CAN1_Vote2_bc0_TAG]
  COMM Task - Vote2/2(Receive CAN1) -> [receive_CAN1_Vote2_bc0_TAG]
  COMM Task - Vote2/3(Send CAN2) -> [send_CAN2_Vote2_bc0_TAG]
  AND8/1 -> COMP Task - Vote2 check/Enable
  GreaterThan25/1 -> AND10/2
  GreaterThan24/1 -> AND10/1
  Sum12/1 -> GreaterThan25/2
  Constant10/1 -> Sum12/2
  Constant9/1 -> COMM Task - Vote3/1(Time Mark), Sum12/1, GreaterThan24/2
  GreaterThan21/1 -> AND11/2
  Sum13/1 -> GreaterThan21/2
  GreaterThan20/1 -> AND11/1
  Constant22/1 -> Sum13/2
  Constant23/1 -> COMP Task - Vote3 check/1(Time_Mark), GreaterThan20/2, Sum13/1
  AND12/1 -> COMP Task - Vote3 Count/Enable
  Constant8/1 -> COMP Task - Vote3 Count/1(Time Mark), Sum11/1, GreaterThan22/2
  Constant7/1 -> Sum11/2
  GreaterThan22/1 -> AND12/1
  Sum11/1 -> GreaterThan23/2
  GreaterThan23/1 -> AND12/2
  COMM Task - Vote3/1(Send CAN1) -> [send_CAN1_Vote3_bc0_TAG]
  COMM Task - Vote3/2(Receive CAN1) -> [receive_CAN1_Vote3_bc0_TAG]
  COMM Task - Vote3/3(Send CAN2) -> [send_CAN2_Vote3_bc0_TAG]
  COMM Task - Vote3/4(Receive CAN2) -> [receive_CAN2_Vote3_bc0_TAG]
  AND10/1 -> COMM Task - Vote3/Enable
  AND11/1 -> COMP Task - Vote3 check/Enable
  GreaterThan27/1 -> AND13/2
  Sum14/1 -> GreaterThan27/2
  GreaterThan26/1 -> AND13/1
  Constant11/1 -> Sum14/2
  Constant12/1 -> COMP Task - Check Timeouts/1(Time_Mark), GreaterThan26/2, Sum14/1
  AND13/1 -> COMP Task - Check Timeouts/Enable
  AND14/1 -> COMP Task - New Master/Enable
  Constant14/1 -> COMP Task - New Master/1(Time_Mark), Sum15/1, GreaterThan28/2
  Constant13/1 -> Sum15/2
  GreaterThan28/1 -> AND14/1
  Sum15/1 -> GreaterThan29/2
  GreaterThan29/1 -> AND14/2
  GreaterThan31/1 -> AND15/2
  Sum16/1 -> GreaterThan31/2
  GreaterThan30/1 -> AND15/1
  Constant24/1 -> Sum16/2
  Constant25/1 -> COMP Task - Reset Variables BC0/1(Time_Mark), GreaterThan30/2, Sum16/1
  AND15/1 -> COMP Task - Reset Variables BC0/Enable
  Data Store Read8/1 -> GreaterThan21/1, GreaterThan20/1, GreaterThan22/1, GreaterThan23/1, GreaterThan32/1, GreaterThan33/1, GreaterThan31/1, GreaterThan30/1, GreaterThan28/1, GreaterThan29/1, GreaterThan27/1, GreaterThan26/1, GreaterThan25/1, GreaterThan24/1, GreaterThan17/1, GreaterThan16/1, GreaterThan14/1, GreaterThan15/1, GreaterThan18/1, GreaterThan19/1, GreaterThan12/1, GreaterThan13/1, GreaterThan11/1, GreaterThan10/1, GreaterThan9/1, GreaterThan8/1, GreaterThan6/1, GreaterThan7/1, GreaterThan4/1, GreaterThan5/1, GreaterThan2/1, GreaterThan3/1, GreaterThan/1, GreaterThan1/1
  AND16/1 -> COMP Task - Reset Board/Enable
  Constant31/1 -> COMP Task - Reset Board/1(Time_Mark), Sum17/1, GreaterThan32/2
  Constant30/1 -> Sum17/2
  GreaterThan32/1 -> AND16/1
  Sum17/1 -> GreaterThan33/2
  GreaterThan33/1 -> AND16/2
  Data Store Read11/1 -> NOT2/1
  NOT2/1 -> AND17/2
  AND17/1 -> COMM Task - Sync bc 0/Enable
  Data Store Read6/1 -> NOT1/1
  NOT1/1 -> AND18/2
  AND1/1 -> AND18/1
  AND18/1 -> COMP Task - Sync bc0 check/Enable
  Data Store Read7/1 -> NOT3/1
  NOT3/1 -> AND19/2
  AND2/1 -> AND19/1
  AND19/1 -> COMP Task - Update LT/Enable
  COMM Task - Vote2/4(Receive CAN2) -> [receive_CAN2_Vote2_bc0_TAG]
  Constant34/1 -> COMP Task - Update LT/2(Time_Mark_2)

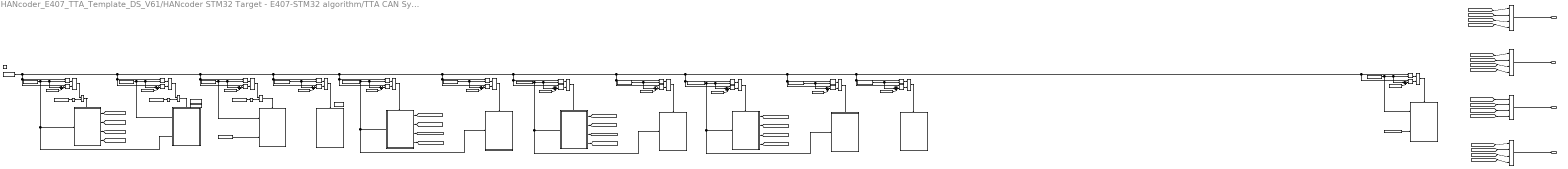
== system HANcoder_E407_TTA_Template_DS_V61/HANcoder STM32 Target - E407-STM32 algorithm/TTA CAN System/TTA System/Matrix Cycle Manager/Controller Matrix Cycle/controller basic cycle 1 ==
  note: Output Send_Message
      | Send: 1
      | Do not send: 0
  note: Output Receive_Message
      | Receive: 1
      | Do not receive: 0
  note: Output Receive_Message
      | Receive: 1
      | Do not receive: 0
  note: Output Send_Message
      | Send: 1
      | Do not send: 0
  note: COMM - TW check
  note: COMP - TW check
  note: Local Time still not updated
  note: COMP - TW check
  note: Local Time still not updated
  note: Local Time still not updated
  note: COMP - TW check
  note: COMM - TW check
  note: COMP - TW check
  note: COMM - TW check
  note: COMP - TW check
  note: COMP - TW check
  note: COMP - TW check
  note: COMM - TW check
  note: COMP - TW check
  Enable : EnablePort
  AND{,1..10,17..20} (15 alike) : Logic  IconShape=distinctive  AllPortsSameDT=off  OutDataTypeStr=boolean
  COMM Task - PotValue board 1 : Subsystem
  COMM Task - PotValue board 2 : Subsystem
  COMM Task - PotValue board 3 : Subsystem
  COMM Task - Sync bc 1 : Subsystem
  COMP Task - Potentiometer Voting : Subsystem
  COMP Task - Reset Variables BC1 : Subsystem
  COMP Task - Rx_PotValues1_check : Subsystem
  COMP Task - Rx_PotValues1_check2 : Subsystem
  COMP Task - Rx_PotValues2_check : Subsystem
  COMP Task - Rx_PotValues3_check : Subsystem
  COMP Task - Sync bc1 check : Subsystem
  COMP Task - Update LT1 : Subsystem
  Constant : Constant  Value=TM_COMM_Sync
  Constant{1,9,18,22} (4 alike) : Constant  Value=COMM_Period
  Constant{2..3,7,10,13,15,21,24} (8 alike) : Constant  Value=COMP_duration
  Constant11 : Constant  Value=TM_COMM_PotValue2
  Constant12 : Constant  Value=TM_Check_PotValue2
  Constant14 : Constant  Value=TM_ReadPot
  Constant16 : Constant  Value=TM_Reset_Var_bc1
  Constant17 : Constant  Value=TM_Update_LT_2
  Constant19 : Constant  Value=TM_COMM_PotValue3
  Constant20 : Constant  Value=TM_Check_PotValue3
  Constant23 : Constant  Value=TM_PotVote
  Constant4 : Constant  Value=TM_Update_LT
  Constant41 : Constant  Value=TM_Reset_Var_bc1_2
  Constant5 : Constant  Value=TM_COMM_PotValue1
  Constant6 : Constant  Value=TM_Check_Sync
  Constant8 : Constant  Value=TM_Check_PotValue1
  Data Store Memory : DataStoreMemory  DataStoreName=OwnPot  WriteAfterWriteMsg=warning  ShowAdditionalParam=off
  Data Store Memory11 : DataStoreMemory  DataStoreName=Msg_Rx  ReadBeforeWriteMsg=warning  WriteAfterWriteMsg=warning  WriteAfterReadMsg=warning  ShowAdditionalParam=off  OutDataTypeStr=Bus: msg_buffer_type
  Data Store Memory8 : DataStoreMemory  DataStoreName=new_msg_Rx  ReadBeforeWriteMsg=warning  WriteAfterWriteMsg=warning  WriteAfterReadMsg=warning  ShowAdditionalParam=off
  Data Store Read1 : DataStoreRead  DataStoreName=Local_Ticks  IndexOptions=Index vector (dialog)  Indices=1  OutputSizes=1
  Data Store Read11 : DataStoreRead  DataStoreName=BC1_Sync_processed  IndexOptions=Index vector (dialog)  Indices=1  OutputSizes=1
  Data Store Read6 : DataStoreRead  DataStoreName=BC1_Sync_processed  IndexOptions=Index vector (dialog)  Indices=1  OutputSizes=1
  Data Store Read7 : DataStoreRead  DataStoreName=BC1_Sync_processed  IndexOptions=Index vector (dialog)  Indices=1  OutputSizes=1
  GreaterThan{,2,4,6,8,10,12,14,16,18,20,34} (12 alike) : RelationalOperator  OutDataTypeStr=boolean  RndMeth=Simplest  InputSameDT=off
  GreaterThan{1,3,5,7,9,11,13,15,17,19,21,35} (12 alike) : RelationalOperator  Operator=<  OutDataTypeStr=boolean  RndMeth=Simplest  InputSameDT=off
  NOT2 : Logic  Operator=NOT  IconShape=distinctive  AllPortsSameDT=off  OutDataTypeStr=boolean
  NOT4 : Logic  Operator=NOT  IconShape=distinctive  AllPortsSameDT=off  OutDataTypeStr=boolean
  NOT5 : Logic  Operator=NOT  IconShape=distinctive  AllPortsSameDT=off  OutDataTypeStr=boolean
  OR{,1..3} (4 alike) : Logic  Operator=OR  Inputs=4  IconShape=distinctive  AllPortsSameDT=off  OutDataTypeStr=boolean
  Sum{1..11,18} (12 alike) : Sum  Inputs=|++
  Send_Message_CAN1 : Outport  OutputWhenDisabled=reset  InitialOutput=0  VectorParamsAs1DForOutWhenUnconnected=off
  Send_Message_CAN2 : Outport  Port=2  OutputWhenDisabled=reset  InitialOutput=0  VectorParamsAs1DForOutWhenUnconnected=off
  Receive_Message_CAN1 : Outport  Port=3  OutputWhenDisabled=reset  InitialOutput=0  VectorParamsAs1DForOutWhenUnconnected=off
  Receive_Message_CAN2 : Outport  Port=4  OutputWhenDisabled=reset  InitialOutput=0  VectorParamsAs1DForOutWhenUnconnected=off
  wires:
  Constant1/1 -> Sum4/2
  COMM Task - Sync bc 1/1(Send CAN1) -> [send_CAN1_Sync_bc1_TAG]
  COMM Task - Sync bc 1/2(Receive CAN1) -> [receive_CAN1_Sync_bc1_TAG]
  COMM Task - Sync bc 1/4(Receive CAN2) -> [receive_CAN2_Sync_bc1_TAG]
  AND19/1 -> COMP Task - Update LT1/Enable
  NOT2/1 -> AND18/2
  Data Store Read7/1 -> NOT5/1
  GreaterThan4/1 -> AND2/1
  AND18/1 -> COMP Task - Sync bc1 check/Enable
  AND1/1 -> AND18/1
  Data Store Read11/1 -> NOT4/1
  AND17/1 -> COMM Task - Sync bc 1/Enable
  AND2/1 -> AND19/1
  Data Store Read6/1 -> NOT2/1
  NOT4/1 -> AND17/2
  GreaterThan1/1 -> AND/2
  GreaterThan/1 -> AND/1
  Constant/1 -> COMP Task - Sync bc1 check/2(TM_COMM), COMM Task - Sync bc 1/1(Time Mark), Sum4/1, GreaterThan/2
  AND/1 -> AND17/1
  Constant3/1 -> Sum2/2
  Constant4/1 -> COMP Task - Update LT1/1(Time_Mark), Sum2/1, GreaterThan4/2
  Sum4/1 -> GreaterThan1/2
  GreaterThan2/1 -> AND1/1
  GreaterThan3/1 -> AND1/2
  Constant2/1 -> Sum1/2
  Constant6/1 -> COMP Task - Sync bc1 check/1(Time_Mark), GreaterThan2/2, Sum1/1
  Sum1/1 -> GreaterThan3/2
  COMM Task - Sync bc 1/3(Send CAN2) -> [send_CAN2_Sync_bc1_TAG]
  NOT5/1 -> AND19/2
  Sum2/1 -> GreaterThan5/2
  GreaterThan5/1 -> AND2/2
  GreaterThan35/1 -> AND20/2
  Constant16/1 -> Sum18/1, GreaterThan34/2, COMP Task - Reset Variables BC1/1(Time_Mark)
  Constant15/1 -> Sum18/2
  Sum18/1 -> GreaterThan35/2
  GreaterThan34/1 -> AND20/1
  AND20/1 -> COMP Task - Reset Variables BC1/Enable
  Constant17/1 -> COMP Task - Update LT1/2(Time_Mark_2)
  Constant41/1 -> COMP Task - Reset Variables BC1/2(Time_Mark_2)
  COMM Task - PotValue board 1/3(Send CAN2) -> [send_CAN2_PotValue1_bc1_TAG]
  AND3/1 -> COMM Task - PotValue board 1/Enable
  COMM Task - PotValue board 1/2(Receive CAN1) -> [receive_CAN1_PotValue1_bc1_TAG]
  COMM Task - PotValue board 1/1(Send CAN1) -> [send_CAN1_PotValue1_bc1_TAG]
  GreaterThan7/1 -> AND3/2
  Constant18/1 -> Sum3/2
  Sum3/1 -> GreaterThan7/2
  GreaterThan6/1 -> AND3/1
  Constant5/1 -> Sum3/1, GreaterThan6/2, COMP Task - Rx_PotValues1_check/1(TM_COMM), COMM Task - PotValue board 1/1(Time Mark)
  COMM Task - PotValue board 1/4(Receive CAN2) -> [receive_CAN2_PotValue1_bc1_TAG]
  Constant10/1 -> Sum6/2
  Sum6/1 -> GreaterThan11/2
  GreaterThan11/1 -> AND5/2
  AND5/1 -> COMP Task - Rx_PotValues1_check/Enable
  Constant8/1 -> Sum6/1, GreaterThan10/2
  GreaterThan10/1 -> AND5/1
  OR/1 -> Send_Message_CAN1/1
  [send_CAN1_Sync_bc1_TAG] -> OR/1
  [send_CAN1_PotValue1_bc1_TAG] -> OR/2
  OR1/1 -> Send_Message_CAN2/1
  [send_CAN2_Sync_bc1_TAG] -> OR1/1
  [send_CAN2_PotValue1_bc1_TAG] -> OR1/2
  OR2/1 -> Receive_Message_CAN1/1
  [receive_CAN1_Sync_bc1_TAG] -> OR2/1
  [receive_CAN1_PotValue1_bc1_TAG] -> OR2/2
  OR3/1 -> Receive_Message_CAN2/1
  [receive_CAN2_Sync_bc1_TAG] -> OR3/1
  [receive_CAN2_PotValue1_bc1_TAG] -> OR3/2
  Constant12/1 -> Sum7/1, GreaterThan8/2
  COMM Task - PotValue board 2/1(Send CAN1) -> [send_CAN1_PotValue2_bc1_TAG]
  GreaterThan8/1 -> AND6/1
  AND4/1 -> COMM Task - PotValue board 2/Enable
  Constant7/1 -> Sum7/2
  COMM Task - PotValue board 2/4(Receive CAN2) -> [receive_CAN2_PotValue2_bc1_TAG]
  Constant11/1 -> Sum5/1, GreaterThan12/2, COMP Task - Rx_PotValues2_check/1(TM_COMM), COMM Task - PotValue board 2/1(Time Mark)
  GreaterThan9/1 -> AND6/2
  GreaterThan12/1 -> AND4/1
  Sum7/1 -> GreaterThan9/2
  AND6/1 -> COMP Task - Rx_PotValues2_check/Enable
  Sum5/1 -> GreaterThan13/2
  COMM Task - PotValue board 2/3(Send CAN2) -> [send_CAN2_PotValue2_bc1_TAG]
  Constant9/1 -> Sum5/2
  COMM Task - PotValue board 2/2(Receive CAN1) -> [receive_CAN1_PotValue2_bc1_TAG]
  GreaterThan13/1 -> AND4/2
  AND7/1 -> COMP Task - Rx_PotValues1_check2/Enable
  GreaterThan14/1 -> AND7/1
  Constant14/1 -> Sum8/1, GreaterThan14/2
  GreaterThan15/1 -> AND7/2
  Sum8/1 -> GreaterThan15/2
  Constant13/1 -> Sum8/2
  [receive_CAN2_PotValue2_bc1_TAG] -> OR3/3
  [receive_CAN1_PotValue2_bc1_TAG] -> OR2/3
  [send_CAN2_PotValue2_bc1_TAG] -> OR1/3
  [send_CAN1_PotValue2_bc1_TAG] -> OR/3
  COMM Task - PotValue board 3/1(Send CAN1) -> [send_CAN1_PotValue3_bc1_TAG]
  GreaterThan19/1 -> AND9/2
  Constant19/1 -> Sum9/1, GreaterThan16/2, COMP Task - Rx_PotValues3_check/1(TM_COMM), COMM Task - PotValue board 3/1(Time Mark)
  GreaterThan17/1 -> AND8/2
  Constant21/1 -> Sum10/2
  COMM Task - PotValue board 3/3(Send CAN2) -> [send_CAN2_PotValue3_bc1_TAG]
  AND8/1 -> COMM Task - PotValue board 3/Enable
  Sum9/1 -> GreaterThan17/2
  Constant22/1 -> Sum9/2
  AND9/1 -> COMP Task - Rx_PotValues3_check/Enable
  GreaterThan18/1 -> AND9/1
  Constant20/1 -> Sum10/1, GreaterThan18/2
  Sum10/1 -> GreaterThan19/2
  COMM Task - PotValue board 3/2(Receive CAN1) -> [receive_CAN1_PotValue3_bc1_TAG]
  GreaterThan16/1 -> AND8/1
  COMM Task - PotValue board 3/4(Receive CAN2) -> [receive_CAN2_PotValue3_bc1_TAG]
  [receive_CAN2_PotValue3_bc1_TAG] -> OR3/4
  [receive_CAN1_PotValue3_bc1_TAG] -> OR2/4
  [send_CAN2_PotValue3_bc1_TAG] -> OR1/4
  [send_CAN1_PotValue3_bc1_TAG] -> OR/4
  AND10/1 -> COMP Task - Potentiometer Voting/Enable
  Sum11/1 -> GreaterThan21/2
  Constant24/1 -> Sum11/2
  GreaterThan20/1 -> AND10/1
  Data Store Read1/1 -> GreaterThan14/1, GreaterThan15/1, GreaterThan7/1, GreaterThan6/1, GreaterThan10/1, GreaterThan11/1, GreaterThan12/1, GreaterThan13/1, GreaterThan8/1, GreaterThan9/1, GreaterThan16/1, GreaterThan17/1, GreaterThan18/1, GreaterThan19/1, GreaterThan20/1, GreaterThan21/1, GreaterThan35/1, GreaterThan34/1, GreaterThan4/1, GreaterThan5/1, GreaterThan2/1, GreaterThan3/1, GreaterThan/1, GreaterThan1/1
  Constant23/1 -> Sum11/1, GreaterThan20/2
  GreaterThan21/1 -> AND10/2
